simulink model "VtP_mod2_SilvaSteensgaard"  (Simulink 7.9)
settings: Solver=ode45  StartTime=0.0  StopTime=simu.trantime  RelTol=1e-3
undefined symbols (not defined in the file): dc, Fs, mod, OSR, sinamp, sinfreq
libraries: dspsigops x4, dspsigattribs x2, dsparch4 x1, simulink x1, commsrccod2 x1, dspmtrx3 x1, commblksprivate x1, dspsrcs4 x1
settings Model: Creator=Isacco Arnaldi  LastModifiedBy=Arnaldi Isacco
settings SolverCC: ZcThreshold=1e-3  ZeroCrossAlgorithm=Adaptive  AutoInsertRateTranBlk=on
settings DataIOCC: MaxDataPoints=50000  SaveOutput=off  SignalLogging=off  DSMLogging=off  SaveTime=off
settings DebuggingCC: StrictBusMsg=Warning
settings CodeAppCC: CustomSymbolStrType=$N$R$M_T
settings GRTTargetCC: CombineOutputUpdateFcns=off  GRTInterface=on

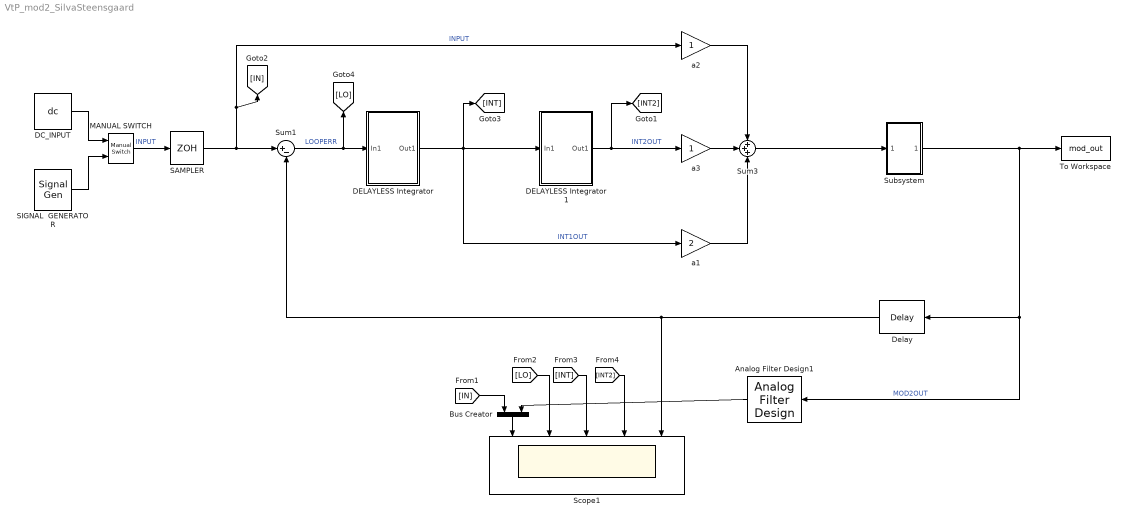
== system VtP_mod2_SilvaSteensgaard ==
  Analog Filter Design1 : dsparch4/Analog Filter Design  method=Butterworth  filttype=Lowpass  N=8  Wlo=pi*(Fs/OSR)  Whi=80  Rp=2  Rs=40
  Bus Creator : BusCreator  Inputs=2
  DC_INPUT : Constant  Value=dc  VectorParams1D=off  OutDataTypeStr=double  SampleTime=1/Fs
  DELAYLESS Integrator : Subsystem
  DELAYLESS Integrator1 : Subsystem
  Delay : dspsigops/Delay  InputProcessing=Inherited (this choice will be removed - see release notes)  dly_unit=Samples  delay=1  ic_detail=off  dif_ic_for_ch=off  dif_ic_for_dly=off  ic=0  reset_popup=None
  MANUAL SWITCH : simulink/Signal Routing/Manual Switch  sw=0  action=0  varsize=off
      settings: AttributesFormatString=Double click to\nselect the desired\ninput
  SAMPLER : ZeroOrderHold  SampleTime=1/Fs
  SIGNAL  GENERATOR : SignalGenerator  Amplitude=sinamp  Frequency=sinfreq  VectorParams1D=off
  Scope1 : Scope  NumInputPorts=5
      settings: TimeRange=2.089895171320487e-05  YMin=-1.1~-0.6~-0.6~-0.3~-5  YMax=1.1~1.6~1.6~0.1~5
  Subsystem : Subsystem
  Sum1 : Sum  Inputs=|+-
      settings: AttributesFormatString=Modulator Input\nLoop Error (input - fbk)
  Sum3 : Sum  Inputs=+++
  To Workspace : ToWorkspace  VariableName=mod_out  SampleTime=-1
      settings: AttributesFormatString=Export output to\nworkspace for\npost-processing
  a1 : Gain  Gain=2
  a2 : Gain
  a3 : Gain
  wires:
  Sum1/1 -> DELAYLESS Integrator/1(In1), [LO]  "LOOPERR"
  DC_INPUT/1 -> MANUAL SWITCH/1
  SIGNAL  GENERATOR/1 -> MANUAL SWITCH/2
  Sum3/1 -> Subsystem/1(In1)
  Subsystem/1(Out1) -> To Workspace/1, Delay/1, Analog Filter Design1/1  "MOD2OUT"
  DELAYLESS Integrator/1(Out1) -> a1/1, DELAYLESS Integrator1/1(In1), [INT]  "INT1OUT"
  DELAYLESS Integrator1/1(Out1) -> a3/1, [INT2]  "INT2OUT"
  a1/1 -> Sum3/3
  a2/1 -> Sum3/1
  a3/1 -> Sum3/2
  Delay/1 -> Sum1/2, Scope1/5
  SAMPLER/1 -> Sum1/1, a2/1, [IN]  "INPUT"
  MANUAL SWITCH/1 -> SAMPLER/1  "INPUT"
  [IN] -> Bus Creator/1
  Bus Creator/1 -> Scope1/1
  Analog Filter Design1/1 -> Bus Creator/2
  [LO] -> Scope1/2
  [INT] -> Scope1/3
  [INT2] -> Scope1/4

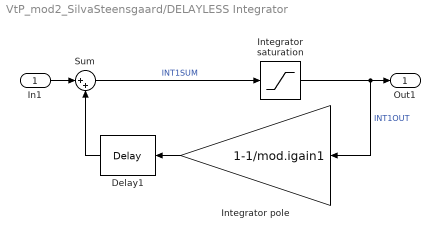
== system VtP_mod2_SilvaSteensgaard/DELAYLESS Integrator ==
  In1 : Inport
  Delay1 : dspsigops/Delay  InputProcessing=Inherited (this choice will be removed - see release notes)  dly_unit=Samples  delay=1  ic_detail=off  dif_ic_for_ch=off  dif_ic_for_dly=off  ic=0  reset_popup=None
  Integrator pole : Gain  Gain=1-1/mod.igain1
      settings: AttributesFormatString=(model finite dc gain)
  Integrator saturation : Saturate  UpperLimit=mod.isat1  LowerLimit=-(mod.isat1)
  Sum : Sum  Inputs=|++  SampleTime=1/Fs
      settings: AttributesFormatString=Integrator summer
  Out1 : Outport
  wires:
  Integrator saturation/1 -> Integrator pole/1, Out1/1  "INT1OUT"
  In1/1 -> Sum/1
  Integrator pole/1 -> Delay1/1
  Delay1/1 -> Sum/2
  Sum/1 -> Integrator saturation/1  "INT1SUM"

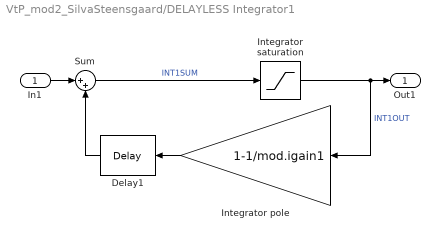
== system VtP_mod2_SilvaSteensgaard/DELAYLESS Integrator1 ==
  In1 : Inport
  Delay1 : dspsigops/Delay  InputProcessing=Inherited (this choice will be removed - see release notes)  dly_unit=Samples  delay=1  ic_detail=off  dif_ic_for_ch=off  dif_ic_for_dly=off  ic=0  reset_popup=None
  Integrator pole : Gain  Gain=1-1/mod.igain1
      settings: AttributesFormatString=(model finite dc gain)
  Integrator saturation : Saturate  UpperLimit=mod.isat1  LowerLimit=-(mod.isat1)
  Sum : Sum  Inputs=|++  SampleTime=1/Fs
      settings: AttributesFormatString=Integrator summer
  Out1 : Outport
  wires:
  Integrator saturation/1 -> Integrator pole/1, Out1/1  "INT1OUT"
  In1/1 -> Sum/1
  Integrator pole/1 -> Delay1/1
  Delay1/1 -> Sum/2
  Sum/1 -> Integrator saturation/1  "INT1SUM"

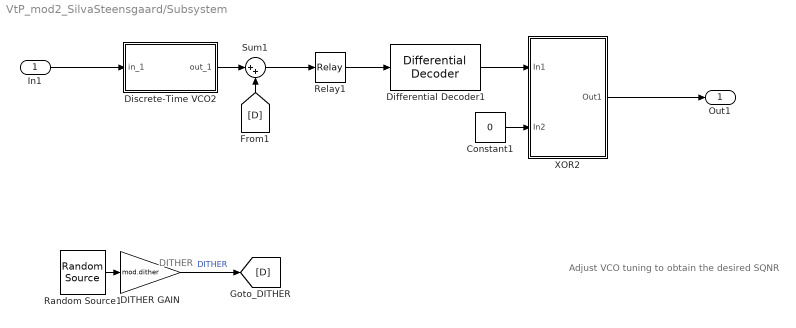
== system VtP_mod2_SilvaSteensgaard/Subsystem ==
  note: DITHER
  note: Adjust VCO tuning to obtain the desired SQNR
  In1 : Inport
  Constant1 : Constant  Value=0  VectorParams1D=off  OutDataTypeStr=boolean  SampleTime=1/Fs
  DITHER GAIN : Gain  Gain=mod.dither  SampleTime=1/Fs
  Differential Decoder1 : commsrccod2/Differential Decoder  InitCond=0
  Discrete-Time VCO2 : Subsystem  AncestorBlock=commsynccomp2/Discrete-Time VCO  mask(Discrete-Time VCO){Ac=sinamp*2, Fc=Fs/128, Kc=sinfreq*3, Ph=0, ts=1/Fs}
      mask prompts: Ac "Output amplitude (V):"; Fc "Quiescent frequency (Hz):"; Kc "Input sensitivity (Hz/V):"; Ph "Initial phase (rad):"; ts "Sample time (s):"
      mask help: Generate a discrete-time output signal whose frequency changes in response to the amplitude variations of the input signal. The input signal must be a scalar.
      mask init:
      | if ( (length(Ac)~=1) || (length(Fc)~=1) || (length(Kc)~=1) || (length(Ph)~=1) || (length(ts)~=1) ) 
      | 	error('commblks:DiscTimeVCO:InvalidMaskParams',...
      |           'Mask parameters must be scalar values.');
      | end
      | FcRadians = 2*pi*Fc;
      | KcRadPerV = 2*pi*Kc;
      mask Help: helpview(commbhelp)
      mask Display: disp('Discrete-Time\nVCO')
  Random Source1 : dspsrcs4/Random Source  SrcType=Uniform  NormMethod=Ziggurat  CltLength=12  MinVal=-1  MaxVal=1  MeanVal=0  VarVal=1  RepMode=Not repeatable  rawSeed=1  IsInherit=off  SampMode=Discrete  SampTime=1/Fs  SampFrame=1  DataType=Double  OutComplex=Real
  Relay1 : Relay  SampleTime=1/Fs
  Sum1 : Sum  Inputs=|++  SampleTime=1/Fs
  XOR2 : Subsystem
  Out1 : Outport
  wires:
  XOR2/1(Out1) -> Out1/1
  In1/1 -> Discrete-Time VCO2/1(in_1)
  Random Source1/1 -> DITHER GAIN/1
  DITHER GAIN/1 -> [D]  "DITHER"
  Relay1/1 -> Differential Decoder1/1
  Constant1/1 -> XOR2/2(In2)
  Differential Decoder1/1 -> XOR2/1(In1)
  [D] -> Sum1/2
  Discrete-Time VCO2/1(out_1) -> Sum1/1
  Sum1/1 -> Relay1/1

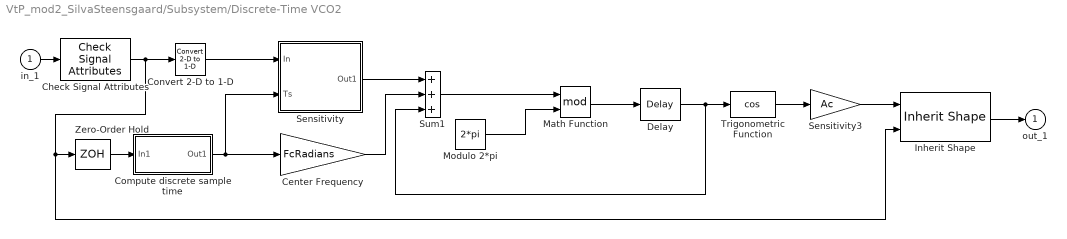
== system VtP_mod2_SilvaSteensgaard/Subsystem/Discrete-Time VCO2 ==
  in_1 : Inport
  Center Frequency : Gain  Gain=FcRadians  ParamDataTypeStr=float('double')  OutDataTypeStr=Inherit: Inherit via back propagation  RndMeth=Nearest  SampleTime=ts  SaturateOnIntegerOverflow=on
  Check Signal Attributes : dspsigattribs/Check Signal Attributes  SigAttribCheckMethod=Does not match attributes exactly  Complexity=Ignore  Frame=Ignore  DimsCheckMethod=Is...  Dimensions=Scalar (1-D or 2-D)  DatatypeCheckMethod=Is...  DatatypeGeneral=Floating-point  DtypeFloatSpecific=Any floating-point  DtypeFixedSpecific=Any fixed-point  DtypeIntSpecific=Any integer  SampleMode=Discrete
  Compute discrete sample time : Subsystem
  Convert 2-D to 1-D : dspsigattribs/Convert 2-D to 1-D
  Delay : dspsigops/Delay  InputProcessing=Columns as channels (frame based)  dly_unit=Samples  delay=1  ic_detail=on  dif_ic_for_ch=off  dif_ic_for_dly=off  ic=Ph  reset_popup=None
  Inherit Shape : commblksprivate/Inherit Shape
  Math Function : Math  Operator=mod  SaturateOnIntegerOverflow=on
  Modulo 2*pi : Constant  Value=2*pi  OutDataTypeStr=Inherit: Inherit via back propagation  SampleTime=ts
  Sensitivity : Subsystem
  Sensitivity3 : Gain  Gain=Ac  SaturateOnIntegerOverflow=on  OutDataTypeStr=Inherit: Same as input  ParamDataTypeStr=Inherit: Same as input
  Sum1 : Sum  Inputs=+++  SaturateOnIntegerOverflow=on  InputSameDT=on  OutDataTypeStr=Inherit: Same as first input
  Trigonometric Function : Trigonometry  Operator=cos
  Zero-Order Hold : ZeroOrderHold  SampleTime=ts
  out_1 : Outport  InitialOutput=0
  wires:
  Zero-Order Hold/1 -> Compute discrete sample time/1(In1)
  Sensitivity/1(Out1) -> Sum1/1
  Compute discrete sample time/1(Out1) -> Sensitivity/2(Ts), Center Frequency/1
  Center Frequency/1 -> Sum1/2
  Check Signal Attributes/1 -> Inherit Shape/2, Zero-Order Hold/1, Convert 2-D to 1-D/1
  Trigonometric Function/1 -> Sensitivity3/1
  in_1/1 -> Check Signal Attributes/1
  Math Function/1 -> Delay/1
  Sum1/1 -> Math Function/1
  Modulo 2*pi/1 -> Math Function/2
  Convert 2-D to 1-D/1 -> Sensitivity/1(In)
  Sensitivity3/1 -> Inherit Shape/1
  Inherit Shape/1 -> out_1/1
  Delay/1 -> Trigonometric Function/1, Sum1/3

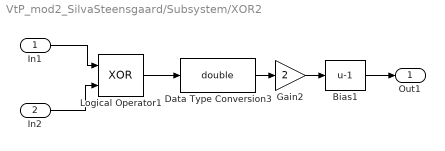
== system VtP_mod2_SilvaSteensgaard/Subsystem/XOR2 ==
  In1 : Inport
  In2 : Inport  Port=2
  Bias1 : Bias  Bias=-1
  Data Type Conversion3 : DataTypeConversion  OutDataTypeStr=double  SampleTime=1/Fs
  Gain2 : Gain  Gain=2  SampleTime=1/Fs
  Logical Operator1 : Logic  Operator=XOR  IconShape=distinctive  AllPortsSameDT=off  OutDataTypeStr=boolean  SampleTime=1/Fs
  Out1 : Outport
  wires:
  Logical Operator1/1 -> Data Type Conversion3/1
  Data Type Conversion3/1 -> Gain2/1
  Gain2/1 -> Bias1/1
  Bias1/1 -> Out1/1
  In2/1 -> Logical Operator1/2
  In1/1 -> Logical Operator1/1

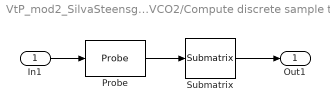
== system VtP_mod2_SilvaSteensgaard/Subsystem/Discrete-Time VCO2/Compute discrete sample time ==
  In1 : Inport
  Probe : Probe  ProbeWidth=off  ProbeComplexSignal=off
  Submatrix : dspmtrx3/Submatrix  RowSpan=One row  RowStartMode=First  RowStartIndex=1  RowEndMode=Last  RowEndIndex=1  ColSpan=One column  ColStartMode=First  ColStartIndex=1  ColEndMode=Last  ColEndIndex=1
  Out1 : Outport
  wires:
  Submatrix/1 -> Out1/1
  In1/1 -> Probe/1
  Probe/1 -> Submatrix/1

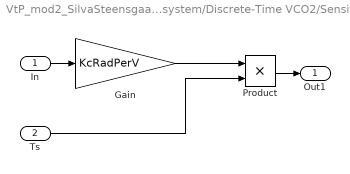
== system VtP_mod2_SilvaSteensgaard/Subsystem/Discrete-Time VCO2/Sensitivity ==
  In : Inport
  Ts : Inport  Port=2
  Gain : Gain  Gain=KcRadPerV  ParamDataTypeStr=float('double')  SaturateOnIntegerOverflow=on  OutDataTypeStr=Inherit: Same as input
  Product : Product  RndMeth=Nearest  SaturateOnIntegerOverflow=on  OutDataTypeStr=Inherit: Same as first input
  Out1 : Outport
  wires:
  Product/1 -> Out1/1
  In/1 -> Gain/1
  Ts/1 -> Product/2
  Gain/1 -> Product/1
